simulink subsystem "baseline_controller"  (R2023b)
settings: Solver=VariableStepAuto  StartTime=0.0  StopTime=10.0  RelTol=1e-3
values from neighbouring files (symbols this model uses):
  K_p = 30    [baseline_controller_parameters.m]
  T_i = 1    [baseline_controller_parameters.m]
undefined symbols (not defined in the file or in its folder): omega_in_max, tau_s
settings Model: Creator=Previ  LastModifiedBy=Previ

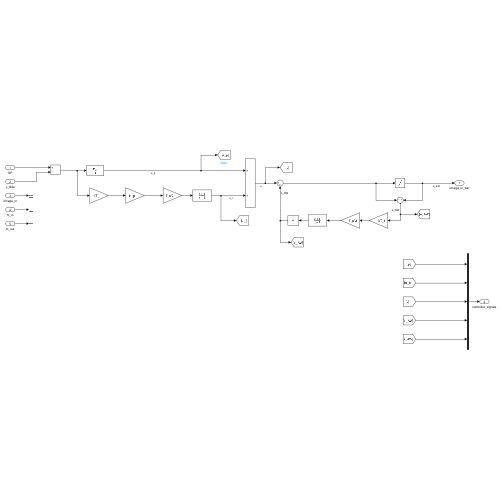
[thumbnail: Simulink's stored preview of the top-level diagram]
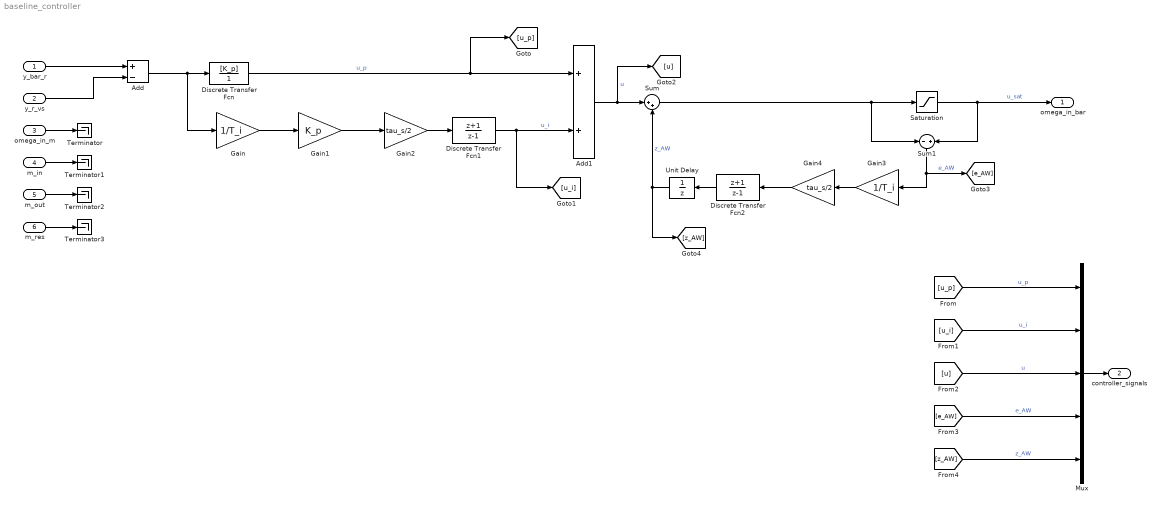
== system baseline_controller ==
  y_bar_r : Inport  PortDimensions=[1, 1]
  y_r_vs : Inport  Port=2  PortDimensions=[1, 1]
  omega_in_m : Inport  Port=3  PortDimensions=[1, 1]
  m_in : Inport  Port=4  PortDimensions=[1, 1]
  m_out : Inport  Port=5  PortDimensions=[1, 1]
  m_res : Inport  Port=6  PortDimensions=[1, 1]
  Add : Sum  Inputs=+-
  Add1 : Sum
  Discrete Transfer Fcn : DiscreteTransferFcn  Numerator=[K_p]  Denominator=[1]
  Discrete Transfer Fcn1 : DiscreteTransferFcn  Numerator=[1 1]  Denominator=[1 -1]
  Discrete Transfer Fcn2 : DiscreteTransferFcn  Numerator=[1 1]  Denominator=[1 -1]
  Gain : Gain  Gain=1/T_i
  Gain1 : Gain  Gain=K_p
  Gain2 : Gain  Gain=tau_s/2
  Gain3 : Gain  Gain=1/T_i
  Gain4 : Gain  Gain=tau_s/2
  Mux : Mux  Inputs=5
  Saturation : Saturate  UpperLimit=omega_in_max  LowerLimit=0
  Sum : Sum  Inputs=|++
  Sum1 : Sum  Inputs=-|+
  Terminator{,1..3} (4 alike) : Terminator
  Unit Delay : UnitDelay  SampleTime=tau_s  HasFrameUpgradeWarning=on
  omega_in_bar : Outport  PortDimensions=[1, 1]
  controller_signals : Outport  Port=2  PortDimensions=[5, 1]
  wires:
  y_r_vs/1 -> Add/2
  m_out/1 -> Terminator2/1
  m_in/1 -> Terminator1/1
  y_bar_r/1 -> Add/1
  omega_in_m/1 -> Terminator/1
  Saturation/1 -> Sum1/2, omega_in_bar/1  "u_sat"
  Mux/1 -> controller_signals/1
  Add/1 -> Gain/1, Discrete Transfer Fcn/1
  Discrete Transfer Fcn1/1 -> [u_i], Add1/2  "u_i"
  Gain2/1 -> Discrete Transfer Fcn1/1
  Gain1/1 -> Gain2/1
  Gain/1 -> Gain1/1
  Discrete Transfer Fcn/1 -> [u_p], Add1/1  "u_p"
  Add1/1 -> [u], Sum/1  "u"
  Sum/1 -> Sum1/1, Saturation/1
  Sum1/1 -> [e_AW], Gain3/1  "e_AW"
  Gain3/1 -> Gain4/1
  Gain4/1 -> Discrete Transfer Fcn2/1
  Discrete Transfer Fcn2/1 -> Unit Delay/1
  Unit Delay/1 -> [z_AW], Sum/2  "z_AW"
  [u_p] -> Mux/1  "u_p"
  [u_i] -> Mux/2  "u_i"
  [u] -> Mux/3  "u"
  [e_AW] -> Mux/4  "e_AW"
  [z_AW] -> Mux/5  "z_AW"
  m_res/1 -> Terminator3/1
